simulink model "Clutchless_P2_Parallel"  (R2017b)
settings: Solver=FixedStepAuto  StartTime=0.0  StopTime=length(Speed)  FixedStep=0.01  MaxStep=0.01  RelTol=1e-3  EnableMultiTasking=on
PostLoadFcn:
  | , if any(exist('dsrtsu_mdlpostloadfcn', 'file') == [2, 3, 6]), try dsrtsu_mdlpostloadfcn('Execute', bdroot); catch fprintf('Error in PostLoadFcn (dsrtsu_mdlpostloadfcn) for model "%s":\n %s\n', bdroot, lasterr); end, end,
undefined symbols (not defined in the file): Actuators, APP1_OOR, APP2_OOR, APP_Mismatch, Brk_Flt, cal, Chassis, ClutchEngag, Clutchless_HSC, eng, Engine, EngineTorqueReal, EngOverTemp, ENGTRQ_MSMCH_Degraded_CP, ENGTRQ_MSMCH_ErrCritical_CP, ENGTRQ_MSMCH_LimpHome_CP, EngTrqMismatch, ess, ESSOverTemp, g, gb, Grade, KeyPos_Flt, lib_Actuators, lib_Chassis, lib_Clutchless_HSC, lib_EMachine_2017a, lib_Sensors_2017a, LossCAN, Machine, MCUOverTemp, mot, MotDirMismatch, motor_Trq, MotOverTemp, MotTrqMismatch, mph2ms, PRNDL_Flt, RegenFault, rho, Sensors, t_amb, time, tloop, veh, Vehicle
libraries: simulink x96, EC2_libraries x6, autolibmappedmotor x3, powerlib_meascontrol x2, CalculationGallon x1, lib_DCDC x1, lib_Differential x1, lib_HVESS x1, lib_Engine x1, lib_OBC x1, Scope_new x1, lib_Transmission x1
(part 6 of 10)

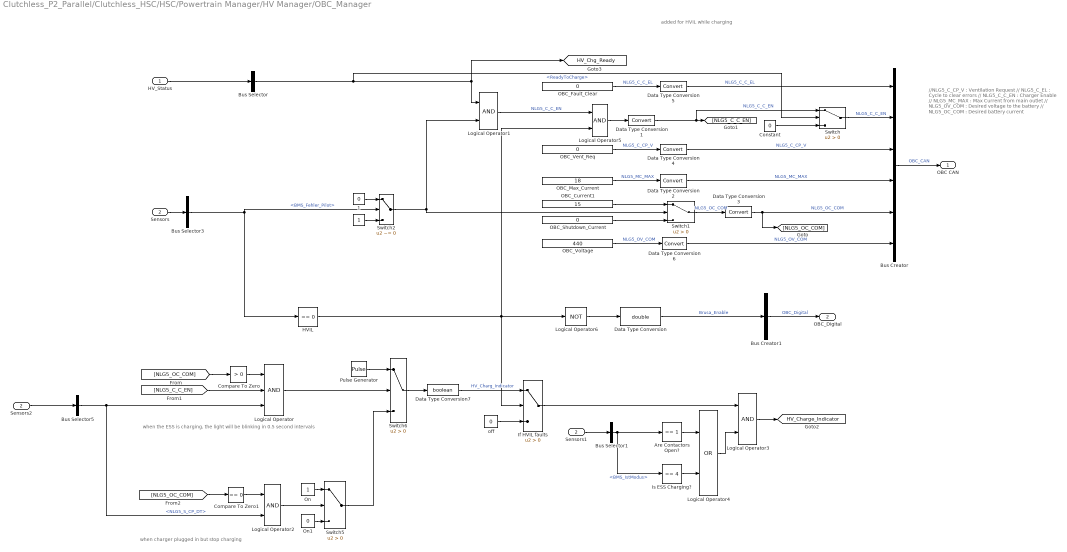
== system Clutchless_P2_Parallel/Clutchless_HSC/HSC/Powertrain Manager/HV Manager/OBC_Manager ==
  note: when the ESS is charging, the light will be blinking in 0.5 second intervals
  note: when charger plugged in but stop charging
  note: //NLG5_C_CP_V : Ventilation Request
      | // NLG5_C_EL : Cycle to clear errors
      | // NLG5_C_C_EN : Charger Enable
      | // NLG5_MC_MAX : Max Current from main outlet
      | // NLG5_OV_COM : Desired voltage to the battery
      | // NLG5_OC_COM : Desired battery current
  note: added for HVIL
      | while charging
  HV_Status : Inport
  Sensors : Inport  Port=2
  " " : Constant
  "   1" : Constant  Value=0
  Are Contactors Open? : simulink/Logic and Bit Operations/Compare To Constant  relop===  const=1  OutDataTypeStr=boolean
  Bus Creator : BusCreator  Inputs=6
  Bus Creator1 : BusCreator  Inputs=1
  Bus Selector : BusSelector  OutputSignals=ReadyToCharge
  Bus Selector1 : BusSelector  OutputSignals=from_CAN.fromHV_CAN.from_BMSHybrid.BMS_HYB_02.BMS_IstModus
  Bus Selector3 : BusSelector  OutputSignals=from_CAN.fromHV_CAN.from_BMSHybrid.BMS_HYB_02.BMS_Fehler_Pilot
  Bus Selector5 : BusSelector  OutputSignals=from_CAN.fromHV_CAN.from_OBC.NLG5_ST.NLG5_S_CP_DT
  Compare To Zero : simulink/Logic and Bit Operations/Compare To Zero  relop=>  OutDataTypeStr=boolean
  Compare To Zero1 : simulink/Logic and Bit Operations/Compare To Zero  relop===  OutDataTypeStr=boolean
  Constant : Constant  Value=0
  Data Type Conversion : DataTypeConversion  OutDataTypeStr=double
  Data Type Conversion{1..6} (6 alike) : DataTypeConversion
  Data Type Conversion7 : DataTypeConversion  OutDataTypeStr=boolean
  HVIL : simulink/Logic and Bit Operations/Compare To Constant  relop===  const=0  OutDataTypeStr=boolean
  If HVIL faults : Switch  Criteria=u2 > Threshold
  Is ESS Charging? : simulink/Logic and Bit Operations/Compare To Constant  relop===  const=4  OutDataTypeStr=boolean
  Logical Operator : Logic  Inputs=3  AllPortsSameDT=off  OutDataTypeStr=boolean
  Logical Operator{1..3,5} (4 alike) : Logic  AllPortsSameDT=off  OutDataTypeStr=boolean
  Logical Operator4 : Logic  Operator=OR  AllPortsSameDT=off  OutDataTypeStr=boolean
  Logical Operator6 : Logic  Operator=NOT  Inputs=3  AllPortsSameDT=off  OutDataTypeStr=boolean
  OBC_Current1 : Constant  Value=15
  OBC_Fault_Clear : Constant  Value=0
  OBC_Max_Current : Constant  Value=18
  OBC_Shutdown_Current : Constant  Value=0
  OBC_Vent_Req : Constant  Value=0
  OBC_Voltage : Constant  Value=440
  On : Constant
  On1 : Constant  Value=0
  Pulse Generator : DiscretePulseGenerator  PulseType=Time based  Period=1  PulseWidth=50
  Sensors1 : InportShadow  Port=2
  Sensors2 : InportShadow  Port=2
  Switch{,1,5..6} (4 alike) : Switch  Criteria=u2 > Threshold
  Switch2 : Switch  Criteria=u2 ~= 0
  off : Constant  Value=0
  OBC CAN : Outport
  OBC_Digital : Outport  Port=2
  tag scope: HV_Charge_Indicator=global, HV_Chg_Ready=global
  wires:
  Sensors2/1 -> Bus Selector5/1
  Switch/1 -> Bus Creator/2  "NLG5_C_C_EN"
  Constant/1 -> Switch/3
  Logical Operator6/1 -> Data Type Conversion/1
  Logical Operator5/1 -> Data Type Conversion1/1
  Logical Operator4/1 -> Logical Operator3/2
  Is ESS Charging?/1 -> Logical Operator4/2
  Bus Selector1/1 -> Are Contactors Open?/1, Is ESS Charging?/1  "<BMS_IstModus>"
  Are Contactors Open?/1 -> Logical Operator4/1
  Sensors1/1 -> Bus Selector1/1
  Logical Operator3/1 -> [HV_Charge_Indicator]
  off/1 -> If HVIL faults/3
  If HVIL faults/1 -> Logical Operator3/1
  HVIL/1 -> Logical Operator5/2, If HVIL faults/2, Logical Operator6/1
  "   1"/1 -> Switch2/1
  " "/1 -> Switch2/3
  Bus Creator1/1 -> OBC_Digital/1  "OBC_Digital"
  Data Type Conversion/1 -> Bus Creator1/1  "Brusa_Enable"
  Bus Selector3/1 -> Switch2/2, HVIL/1  "<BMS_Fehler_Pilot>"
  Bus Selector5/1 -> Logical Operator/3, Logical Operator2/2  "<NLG5_S_CP_DT>"
  Switch6/1 -> Data Type Conversion7/1
  Switch5/1 -> Switch6/3
  On1/1 -> Switch5/3
  On/1 -> Switch5/1
  Logical Operator2/1 -> Switch5/2
  Compare To Zero1/1 -> Logical Operator2/1
  [NLG5_OC_COM] -> Compare To Zero1/1
  Pulse Generator/1 -> Switch6/1
  Logical Operator/1 -> Switch6/2
  [NLG5_C_C_EN] -> Logical Operator/2
  Compare To Zero/1 -> Logical Operator/1
  [NLG5_OC_COM] -> Compare To Zero/1
  Sensors/1 -> Bus Selector3/1
  Bus Creator/1 -> OBC CAN/1  "OBC_CAN"
  HV_Status/1 -> Bus Selector/1
  Bus Selector/1 -> [HV_Chg_Ready], Logical Operator1/1, Switch/2  "<ReadyToCharge>"
  Switch2/1 -> Logical Operator1/2, Switch1/2
  Data Type Conversion2/1 -> Bus Creator/4  "NLG5_MC_MAX"
  Data Type Conversion5/1 -> Bus Creator/1  "NLG5_C_C_EL"
  Data Type Conversion4/1 -> Bus Creator/3  "NLG5_C_CP_V"
  Data Type Conversion6/1 -> Bus Creator/6  "NLG5_OV_COM"
  Data Type Conversion3/1 -> [NLG5_OC_COM], Bus Creator/5  "NLG5_OC_COM"
  OBC_Current1/1 -> Switch1/1
  OBC_Shutdown_Current/1 -> Switch1/3
  Data Type Conversion1/1 -> [NLG5_C_C_EN], Switch/1  "NLG5_C_C_EN"
  Logical Operator1/1 -> Logical Operator5/1  "NLG5_C_C_EN"
  Switch1/1 -> Data Type Conversion3/1  "NLG5_OC_COM"
  OBC_Vent_Req/1 -> Data Type Conversion4/1  "NLG5_C_CP_V"
  OBC_Fault_Clear/1 -> Data Type Conversion5/1  "NLG5_C_C_EL"
  OBC_Max_Current/1 -> Data Type Conversion2/1  "NLG5_MC_MAX"
  OBC_Voltage/1 -> Data Type Conversion6/1  "NLG5_OV_COM"
  Data Type Conversion7/1 -> If HVIL faults/1  "HV_Charg_Indicator"

== system Clutchless_P2_Parallel/Clutchless_HSC/HSC/Powertrain Manager/Thermal Manager/Cooling Fan Manger ==
  Temp : Inport
  Bus Selector : BusSelector  OutputSignals=Temp_Signals.EngCltTmp,Temp_Signals.BMS_Temperatur,Temp_Signals.INV_ElectricMachineTemperature,Temp_Signals.INV_InverterTemperature,VehSpdAvgDrvn,Component_State.SysPwrMd
  Constant : Constant  Value=0
  ESSTargTemp : RelationalOperator  OutDataTypeStr=boolean  RndMeth=Nearest
  EnTargTemp : RelationalOperator  OutDataTypeStr=boolean  RndMeth=Nearest
  EnTargTemp1 : RelationalOperator  Operator=>  OutDataTypeStr=boolean  RndMeth=Nearest
  Fan_Disable : Constant  Value=0
  Fan_Enable : Constant
  Fan_EngTempThrshld : Constant  Value=100
  Fan_EssTempThrshld : Constant  Value=25
  Fan_MCUTempThrshld : Constant  Value=35
  Fan_MotTempThrshld : Constant  Value=35
  Fan_VehSpdThrshld : Constant  Value=10
  InvTargTemp : RelationalOperator  OutDataTypeStr=boolean  RndMeth=Nearest
  InvTargTemp1 : RelationalOperator  Operator=<=  OutDataTypeStr=boolean  RndMeth=Nearest
  Logical Operator : Logic  Operator=OR  Inputs=4  AllPortsSameDT=off  OutDataTypeStr=boolean
  Logical Operator1 : Logic  AllPortsSameDT=off  OutDataTypeStr=boolean
  Logical Operator2 : Logic  AllPortsSameDT=off  OutDataTypeStr=boolean
  MorTargTemp : RelationalOperator  OutDataTypeStr=boolean  RndMeth=Nearest
  Switch : Switch  Criteria=u2 ~= 0
  Fan_control : Outport
  wires:
  Fan_VehSpdThrshld/1 -> InvTargTemp1/2
  Fan_MCUTempThrshld/1 -> InvTargTemp/2
  Fan_MotTempThrshld/1 -> MorTargTemp/2
  Fan_EssTempThrshld/1 -> ESSTargTemp/2
  Fan_EngTempThrshld/1 -> EnTargTemp/2
  InvTargTemp1/1 -> Logical Operator1/2
  Bus Selector/5 -> InvTargTemp1/1  "<VehSpdAvgDrvn>"
  Logical Operator/1 -> Logical Operator1/1
  InvTargTemp/1 -> Logical Operator/4
  MorTargTemp/1 -> Logical Operator/3
  ESSTargTemp/1 -> Logical Operator/2
  EnTargTemp/1 -> Logical Operator/1
  Bus Selector/4 -> InvTargTemp/1  "<INV_InverterTemperature>"
  Bus Selector/3 -> MorTargTemp/1  "<INV_ElectricMachineTemperature>"
  Bus Selector/2 -> ESSTargTemp/1  "<BMS_Temperatur>"
  Bus Selector/1 -> EnTargTemp/1  "<EngCltTmp>"
  Fan_Enable/1 -> Switch/1
  Fan_Disable/1 -> Switch/3
  Switch/1 -> Fan_control/1
  Temp/1 -> Bus Selector/1
  Logical Operator2/1 -> Switch/2
  Logical Operator1/1 -> Logical Operator2/1
  EnTargTemp1/1 -> Logical Operator2/2
  Bus Selector/6 -> EnTargTemp1/1  "<SysPwrMd>"
  Constant/1 -> EnTargTemp1/2

== system Clutchless_P2_Parallel/Clutchless_HSC/HSC/Powertrain Manager/Thermal Manager/ESS Pump Manger ==
  note: If ESS temp>35°，enable pump100 and cooling fan and 2-way valve then enable AC-compressor
      |
      | If 35°>ESStemp≥23°，enable pump100 and cooling fan
      |
      | If 23°>ESS temp disable
      |
      | If 15°>ESS temp, enable heat coolant
  ESS_temp : Inport
  Bus Creator : BusCreator  Inputs=4
  Bus Selector : BusSelector  OutputSignals=Temp_Signals.BMS_Temperatur,Component_State.SysPwrMd
  Chart1 : Stateflow chart  TreatAsAtomicUnit=on
  ESS_Comp_TempThrs : Constant  Value=35
  ESS_Temp_State_1_Thrs : Constant  Value=15
  ESS_Temp_State_2_Thrs : Constant  Value=25
  ESS_Temp_State_3_Thrs : Constant  Value=35
  ESS_Thermal_Control : Outport
  wires:
  Bus Creator/1 -> ESS_Thermal_Control/1
  ESS_Comp_TempThrs/1 -> Chart1/5(ESS_Comp_TempThrs)
  ESS_Temp_State_3_Thrs/1 -> Chart1/4(ESS_Temp_State_3_Thrs)
  ESS_Temp_State_2_Thrs/1 -> Chart1/3(ESS_Temp_State_2_Thrs)
  ESS_Temp_State_1_Thrs/1 -> Chart1/2(ESS_Temp_State_1_Thrs)
  Chart1/3(ESS_val) -> Bus Creator/3  "ESS_val"
  Chart1/2(ESS_pump_control) -> Bus Creator/2  "ESS_pump_control"
  Chart1/1(ESS_comp) -> Bus Creator/1  "ESS_comp"
  Bus Selector/1 -> Chart1/1(ESS_temp), Chart1/6(ESS_CltTemp)  "<BMS_Temperatur>"
  ESS_temp/1 -> Bus Selector/1
  Chart1/4(ESS_comp_Enable) -> Bus Creator/4  "ESS_Comp_Enable"
  Bus Selector/2 -> Chart1/7(SysPowMod)  "<SysPwrMd>"

== system Clutchless_P2_Parallel/Clutchless_HSC/HSC/Powertrain Manager/Thermal Manager/MotInv Pump Manger ==
  MotInv_temp : Inport
  Bus Selector : BusSelector  OutputSignals=Temp_Signals.INV_ElectricMachineTemperature,Temp_Signals.INV_InverterTemperature,Component_State.SysPwrMd
  MCUPump_Manager : Stateflow chart  TreatAsAtomicUnit=on
  MCU_Temp_State_1_Thrs : Constant  Value=30
  MCU_Temp_State_2_Thrs : Constant  Value=50
  Mot_Temp_State_1_Thrs : Constant  Value=30
  Mot_Temp_State_2_Thrs1 : Constant  Value=45
  MotInvpump_control : Outport
  wires:
  MCU_Temp_State_2_Thrs/1 -> MCUPump_Manager/6(Mot_Temp_State_2_Thrs)
  Mot_Temp_State_2_Thrs1/1 -> MCUPump_Manager/5(MCU_Temp_State_2_Thrs)
  Mot_Temp_State_1_Thrs/1 -> MCUPump_Manager/3(MCU_Temp_State_1_Thrs)
  MCU_Temp_State_1_Thrs/1 -> MCUPump_Manager/4(Mot_Temp_State_1_Thrs)
  Bus Selector/2 -> MCUPump_Manager/2(MCU_temp)  "<INV_InverterTemperature>"
  Bus Selector/1 -> MCUPump_Manager/1(Motor_temp)  "<INV_ElectricMachineTemperature>"
  MotInv_temp/1 -> Bus Selector/1
  Bus Selector/3 -> MCUPump_Manager/7(SysPowMod)  "<SysPwrMd>"
  MCUPump_Manager/1(MotInvpump_control) -> MotInvpump_control/1

== system Clutchless_P2_Parallel/Clutchless_HSC/HSC/Powertrain Manager/Torque Distribution/AxlTrq_to_EngTrq ==
  note: //From engine axle torque to engine torque//
  note: check this rate limiter
  In1 : Inport
  Compare To Constant : simulink/Logic and Bit Operations/Compare To Constant  relop===  const=0  OutDataTypeStr=boolean
  Constant1 : Constant  Value=max(gb.plant.init.ratio.map)
  Constant5 : Constant  Value=fd.plant.init.ratio
  Divide1 : Product  Inputs=*//
  Ground : Ground  Commented=on
  Rate Limiter : RateLimiter  RisingSlewLimit=1000  FallingSlewLimit=-2000
  Rate Limiter1 : RateLimiter  Commented=on  RisingSlewLimit=Engine.trq_uprate  FallingSlewLimit=Engine.trq_derate
  Ratio Filter : Subsystem
  Switch : Switch  Criteria=u2 > Threshold
  Terminator : Terminator  Commented=on
  Out1 : Outport
  wires:
  Ground/1 -> Rate Limiter1/1
  Rate Limiter1/1 -> Terminator/1
  Ratio Filter/1(Filtered_Ratio) -> Compare To Constant/1, Switch/3
  Rate Limiter/1 -> Out1/1
  Switch/1 -> Divide1/3
  Constant1/1 -> Switch/1
  Compare To Constant/1 -> Switch/2
  [TransRatio] -> Ratio Filter/1(Ratio)
  Divide1/1 -> Rate Limiter/1
  Constant5/1 -> Divide1/2
  In1/1 -> Divide1/1

== system Clutchless_P2_Parallel/Clutchless_HSC/HSC/Powertrain Manager/Torque Distribution/AxlTrq_to_MotTrq ==
  In1 : Inport
  AxlTrq_to_MtrTrq2 : Subsystem
  MotTrq_LowLim : Constant  Value=-250
  MotTrq_UpLim : Constant  Value=325
  Saturation Dynamic : simulink/Discontinuities/Saturation Dynamic  OutMin=[]  OutMax=[]  OutDataTypeStr=Inherit: Same as second input  OutDataType=fixdt(1, 16)  OutScaling=2^-10  DoSatur=off
  electric machine filter : Subsystem
  Out1 : Outport
  wires:
  Saturation Dynamic/1 -> Out1/1  "MtrTrqCmd_AftSat"
  electric machine filter/1(filtered) -> Saturation Dynamic/2  "MotTrqCmd_BefSat"
  AxlTrq_to_MtrTrq2/1(MtrTrqCmd) -> electric machine filter/1(trq)  "MtrTrqCmd"
  In1/1 -> AxlTrq_to_MtrTrq2/1(In1)
  MotTrq_UpLim/1 -> Saturation Dynamic/1
  MotTrq_LowLim/1 -> Saturation Dynamic/3

== system Clutchless_P2_Parallel/Clutchless_HSC/HSC/Powertrain Manager/Torque Distribution/Rate Limiter Motor1 ==
  In1 : Inport
  Compare To Constant : simulink/Logic and Bit Operations/Compare To Constant  relop===  const=4  OutDataTypeStr=boolean
  Derate_CDCS Mode : Constant  Value=-80
  Derate_Sports Mode : Constant  Value=-150
  Rate Limiter Dynamic : simulink/Discontinuities/Rate Limiter Dynamic
      settings: SourceProductName=Simulink
  Switch : Switch  Criteria=u2 > Threshold
  Switch1 : Switch  Criteria=u2 > Threshold
  Uprate_CDCS Mode : Constant  Value=80
  Uprate_Sports Mode : Constant  Value=100
  Out1 : Outport
  wires:
  Compare To Constant/1 -> Switch/2, Switch1/2
  [mode] -> Compare To Constant/1
  Derate_Sports Mode/1 -> Switch1/1
  Derate_CDCS Mode/1 -> Switch1/3
  Switch1/1 -> Rate Limiter Dynamic/3
  Uprate_CDCS Mode/1 -> Switch/3
  Switch/1 -> Rate Limiter Dynamic/1
  Uprate_Sports Mode/1 -> Switch/1
  Rate Limiter Dynamic/1 -> Out1/1
  In1/1 -> Rate Limiter Dynamic/2

== system Clutchless_P2_Parallel/Clutchless_HSC/HSC/Powertrain Manager/Torque Distribution/RegTrqLimit ==
  MotTrqCmd : Inport
  RPM : Inport  Port=2
  Compare To Constant : simulink/Logic and Bit Operations/Compare To Constant  relop=<=  const=0  OutDataTypeStr=boolean
  Divide : Product  Inputs=**
  Regen Trq Derating : Lookup_n-D  NumberOfTableDimensions=1  BreakpointsForDimension1=[0,200,600,800,1000]  Table=[0,0,0,0.8,1]  ExtrapMethod=Clip  UseLastTableValue=on  InternalRulePriority=Speed  RndMeth=Simplest  InputSameDT=on
  Regen Trq Derating1 : Lookup_n-D  Commented=on  NumberOfTableDimensions=1  BreakpointsForDimension1=[0 200 600 800 1000 1200 12000]  Table=[0 0.05 0.5 0.8 0.95 1 1]  ExtrapMethod=Clip  UseLastTableValue=on  InternalRulePriority=Speed  RndMeth=Simplest  InputSameDT=on
  Switch2 : Switch  Criteria=u2 > Threshold
  Out1 : Outport
  wires:
  Regen Trq Derating/1 -> Divide/1
  Divide/1 -> Switch2/1
  Compare To Constant/1 -> Switch2/2
  MotTrqCmd/1 -> Switch2/3, Divide/2, Compare To Constant/1  "MotTrqCmdIn"
  Switch2/1 -> Out1/1  "MotTrqCmdOut"
  RPM/1 -> Regen Trq Derating/1

== system Clutchless_P2_Parallel/Clutchless_HSC/HSC/Powertrain Manager/Torque Distribution/Select_APP ==
  APP_Select : Constant  Value=0
  Data Type Conversion10 : DataTypeConversion  OutDataTypeStr=boolean
  Derate_APP : Constant  Value=-100
  Rate Limiter Dynamic : simulink/Discontinuities/Rate Limiter Dynamic
      settings: SourceProductName=Simulink
  Switch1 : Switch  Criteria=u2 > Threshold
  Uprate_APP : Constant  Value=80
  EngAppReq : Outport
  wires:
  [EngAppReq] -> Switch1/3
  [AccPos_Perc] -> Switch1/1
  Data Type Conversion10/1 -> Switch1/2
  APP_Select/1 -> Data Type Conversion10/1
  Switch1/1 -> Rate Limiter Dynamic/2  "EngAppReq"
  Rate Limiter Dynamic/1 -> EngAppReq/1  "EngAppReq_Limited"
  Uprate_APP/1 -> Rate Limiter Dynamic/1
  Derate_APP/1 -> Rate Limiter Dynamic/3

== system Clutchless_P2_Parallel/Clutchless_HSC/HSC/Powertrain Manager/Torque Distribution/Sport Mode Enable ==
  In1 : Inport
  Bus Selector5 : BusSelector  OutputSignals=from_Analog.Sport_Mode_SW
  Compare To Constant : simulink/Logic and Bit Operations/Compare To Constant  relop===  const=2  OutDataTypeStr=boolean
  Override Sport Switch : Subsystem
  Sports Mode Logic : Stateflow chart  TreatAsAtomicUnit=on
  Out1 : Outport
  wires:
  In1/1 -> Bus Selector5/1
  Bus Selector5/1 -> Sports Mode Logic/1(Voltage_Input)  "<Sport_Mode_SW>"
  Sports Mode Logic/1(Driver_Mode) -> Compare To Constant/1
  Compare To Constant/1 -> Override Sport Switch/1(In1)
  Override Sport Switch/1(Out1) -> Out1/1

== system Clutchless_P2_Parallel/Clutchless_HSC/HSC/Powertrain Manager/Torque Distribution/Subsystem1 ==
  SoC : Inport
  CS_On : Inport  Port=2
  Constant : Constant
  Sample and Hold1 : dspsigops/Sample and Hold  trig=Rising edge  initCond=0  latchinput=off
  Switch : Switch  Criteria=u2 > Threshold
  Faked_SoC : Outport
  wires:
  SoC/1 -> Sample and Hold1/1
  CS_On/1 -> Switch/2, Sample and Hold1/Trigger
  Switch/1 -> Faked_SoC/1
  Sample and Hold1/1 -> Switch/1
  Constant/1 -> Switch/3

== system Clutchless_P2_Parallel/Clutchless_HSC/HSC/Powertrain Manager/Torque Distribution/Supervisory  Control  Logic/VehReady.CD_Mode.Brake_mode.MotTrqCalc1 ==
  note: Regenerative braking:
      | Regenerative braking should be allowed under specific chassis speed:
      | chas_spd_below_no_regen= 1.5;
      | chas_spd_above_full_regen = 3;
      | ess_soc_above_regen_forbidden = .92;  % ESS SOC above which regen braking is forbidden
      | ess_soc_above_regen_allowed = .9;% ESS SOC above which regen braking is allowed
  BPP : Inport
  VehSpd : Inport  Port=2
  ShftLvrPos : Inport  Port=3
  MotSpeed : Inport  Port=4
  TransRatio : Inport  Port=5
  IntdAxleTrq : Inport  Port=6
  f : TriggerPort  TriggerType=function-call  VariantControl=Variant
      settings: CopyFcn=Stateflow.SLINSF.SimulinkMan.removeBlockPreDeleteFcn  PreDeleteFcn=Stateflow.SLINSF.SimulinkMan.unsafePredeleteFcn
  "% to 1 " : Gain  Gain=1/100
  Constant : Constant  Value=0
  Constant1 : Constant  Value=0
  Constant2 : Constant  Value=fd.plant.init.ratio
  Divide : Product  Inputs=***
  Divide2 : Product  Inputs=***
  Index Vector : MultiPortSwitch  DataPortOrder=Zero-based contiguous  Inputs=5  zeroidx=on
  MinMax : MinMax  Function=max  Inputs=2
  Peak trq max - Regen : Lookup  InputValues=mot.plant.init.regen.trq_max.idx1_spd  Table=mot.plant.init.regen.trq_max.map  LookUpMeth=Interpolation-Use End Values  SaturateOnIntegerOverflow=on
  Regen Trq Derating2 : Lookup_n-D  NumberOfTableDimensions=1  BreakpointsForDimension1=[0 10 11 200]  Table=[0 0.5 1 1]  ExtrapMethod=Clip  UseLastTableValue=on  InternalRulePriority=Speed  RndMeth=Simplest  InputSameDT=on
  Regen_derat_overri : Constant  Value=0
  Regen_derat_value : Constant  Value=0.5
  Switch : Switch  Criteria=u2 > Threshold
  limit to -200Nm : Saturate  UpperLimit=0  LowerLimit=-200
  T : Outport
  wires:
  MinMax/1 -> [TrqCalc]
  IntdAxleTrq/1 -> MinMax/1
  Regen_derat_value/1 -> Switch/1
  Switch/1 -> Divide/3
  Regen_derat_overri/1 -> Switch/2
  Regen Trq Derating2/1 -> Switch/3
  Divide2/1 -> MinMax/2  "motor"
  TransRatio/1 -> Divide2/3
  limit to -200Nm/1 -> Divide2/2
  Constant2/1 -> Divide2/1
  Peak trq max - Regen/1 -> Divide/2
  MotSpeed/1 -> Peak trq max - Regen/1  "RPM"
  [TrqCalc] -> Index Vector/5  "N"
  Constant1/1 -> Index Vector/3  "P"
  Constant/1 -> Index Vector/2  "Between Ranges"
  Index Vector/1 -> T/1
  [TrqCalc] -> Index Vector/6  "D"
  [TrqCalc] -> Index Vector/4  "R"
  ShftLvrPos/1 -> Index Vector/1
  VehSpd/1 -> Regen Trq Derating2/1
  Divide/1 -> limit to -200Nm/1
  "% to 1 "/1 -> Divide/1
  BPP/1 -> "% to 1 "/1

== system Clutchless_P2_Parallel/Clutchless_HSC/HSC/Powertrain Manager/Torque Distribution/Supervisory  Control  Logic/VehReady.CD_Mode.Brake_mode.MotTrqCalc2 ==
  note: Regenerative braking:
      | Regenerative braking should be allowed under specific chassis speed:
      | chas_spd_below_no_regen= 1.5;
      | chas_spd_above_full_regen = 3;
      | ess_soc_above_regen_forbidden = .92;  % ESS SOC above which regen braking is forbidden
      | ess_soc_above_regen_allowed = .9;% ESS SOC above which regen braking is allowed
  ShftLvrPos : Inport
  TransRatio : Inport  Port=2
  f : TriggerPort  TriggerType=function-call  VariantControl=Variant
      settings: CopyFcn=Stateflow.SLINSF.SimulinkMan.removeBlockPreDeleteFcn  PreDeleteFcn=Stateflow.SLINSF.SimulinkMan.unsafePredeleteFcn
  Constant : Constant  Value=0
  Constant1 : Constant  Value=0
  Constant2 : Constant  Value=fd.plant.init.ratio
  Divide2 : Product  Inputs=***
  Idle_torque_Regen : Constant  Value=0
  Index Vector : MultiPortSwitch  DataPortOrder=Zero-based contiguous  Inputs=5  zeroidx=on
  T : Outport
  wires:
  Idle_torque_Regen/1 -> Divide2/2
  Divide2/1 -> [TrqCalc]  "motor"
  TransRatio/1 -> Divide2/3
  Constant2/1 -> Divide2/1
  [TrqCalc] -> Index Vector/5  "N"
  Constant1/1 -> Index Vector/3  "P"
  Constant/1 -> Index Vector/2  "Between Ranges"
  Index Vector/1 -> T/1
  [TrqCalc] -> Index Vector/6  "D"
  [TrqCalc] -> Index Vector/4  "R"
  ShftLvrPos/1 -> Index Vector/1

== system Clutchless_P2_Parallel/Clutchless_HSC/HSC/Powertrain Manager/Torque Distribution/Supervisory  Control  Logic/VehReady.CD_Mode.Drive_mode.EngTrq2EngApp ==
  Trq : Inport
  TransRatio : Inport  Port=2
  f : TriggerPort  TriggerType=function-call  VariantControl=Variant
      settings: CopyFcn=Stateflow.SLINSF.SimulinkMan.removeBlockPreDeleteFcn  PreDeleteFcn=Stateflow.SLINSF.SimulinkMan.unsafePredeleteFcn
  0-100% : Saturate  UpperLimit=100  LowerLimit=0
  Compare To Constant : simulink/Logic and Bit Operations/Compare To Constant  relop===  const=0  OutDataTypeStr=boolean
  Constant1 : Constant  Value=eps
  Constant5 : Constant  Value=fd.plant.init.ratio
  Divide1 : Product  Inputs=*//
  EngTrq2EngAPP : Lookup_n-D  NumberOfTableDimensions=1  BreakpointsForDimension1=[0:1:230]  Table="[-0.950562242591810\t-0.861179388327002\t-0.757792747831397\t-0.640901927898975\t-0.511000095283862\t-0.368573976700328\t-0.214103858822793\t-0.0480635882858183\t0.129079428315885\t0.316864224427463\t0.514836273533913\t0.722547489160089\t0.939556224870697\t1.16542727427030\t1.39973187100331\t1.64204768875400\t1.89195884124648\t2.14905588224475\t2.41293580555262\t2.68320204501379\t2.95946447451180\t3.24133940797003\t3.52844959935174\t3.82042424266002\t4.11689897193784\t4.41751586126800\t4.72192342477317\t5.02977661661586\t5.34073683099846\t5.65447190216317\t5.97065610439209\t6.28897015200715\t6.60910119937013\t6.93074284088268\t7.25359511098630\t7.57736448416234\t7.90176387493200\t8.22651263785634\t8.55133656753627\t8.87596789861257\t9.20014530576584\t9.52361390371657\t9.84612524722509\t10.1674373310916\t10.4873145901561\t10.8055278992985\t11.1218545734385\t11.4360783675358\t11.7479894765898\t12.0573845356398\t12.3640666197649\t12.6678452440843\t12.9685363637566\t13.2659623739808\t13.5599521099953\t13.8503408470787\t14.1369703005491\t14.4196886257647\t14.6983504181235\t14.9728167130634\t15.2429549860620\t15.5086391526369\t15.7697495683456\t16.0261730287853\t16.2778027695931\t16.5245384664460\t16.7662862350608\t17.0029586311942\t17.2344746506427\t17.4607597292427\t17.6817457428705\t17.8973710074422\t18.1075802789137\t18.3123247532808\t18.5115620665792\t18.7052562948843\t18.8933779543117\t19.0759040010164\t19.2528178311935\t19.4241092810781\t19.5897746269448\t19.7498165851084\t19.9042443119232\t20.0530734037837\t20.1963258971241\t20.3340302684184\t20.4662214341804\t20.5929407509641\t20.7142360153630\t20.8301614640105\t20.9407777735800\t21.0461520607847\t21.1463578823776\t21.2414752351516\t21.3315905559394\t21.4167967216136\t21.4971930490867\t21.5728852953111\t21.6439856572787\t21.7106127720217\t21.7728917166119\t21.8309540081611\t21.8849376038208\t21.9349869007824\t21.9812527362772\t22.0238923875764\t22.0630695719909\t22.0989544468717\t22.1317236096093\t22.1615600976344\t22.1886533884173\t22.2131993994684\t22.2354004883376\t22.2554654526151\t22.2736095299306\t22.2900543979538\t22.3050281743942\t22.3187654170013\t22.3315071235641\t22.3435007319120\t22.3550001199137\t22.3662656054781\t22.3775639465539\t22.3891683411296\t22.4013584272335\t22.4144202829338\t22.4286464263386\t22.4443358155959\t22.4617938488934\t22.4813323644587\t22.5032696405595\t22.5279303955028\t22.5556457876361\t22.5867534153463\t22.6215973170604\t22.6605279712450\t22.7039022964069\t22.7520836510924\t22.8054418338880\t22.8643530834197\t22.9292000783536\t23.0003719373956\t23.0782642192915\t23.1632789228268\t23.2558244868269\t23.3563157901571\t23.4651741517227\t23.5828273304686\t23.7097095253797\t23.8462613754808\t23.9929299598362\t24.1501687975506\t24.3184378477682\t24.4982035096730\t24.6899386224892\t24.8941224654804\t25.1112407579505\t25.3417856592430\t25.5862557687413\t25.8451561258686\t26.1189982100880\t26.4082999409026\t26.7135856778550\t27.0353862205281\t27.3742388085443\t27.7306871215661\t28.1052812792955\t28.4985778414748\t28.9111398078859\t29.3435366183506\t29.7963441527305\t30.2701447309271\t30.7655271128819\t31.2830864985759\t31.8234245280303\t32.3871492813060\t32.9748752785038\t33.5872234797643\t34.2248212852680\t34.8883025352352\t35.5783075099261\t36.2954829296408\t37.0404819547192\t37.8139641855409\t38.6165956625258\t39.4490488661331\t40.3120027168621\t41.2061425752523\t42.1321602418824\t43.0907539573713\t44.0826284023780\t45.1084946976008\t46.1690704037782\t47.2650795216887\t48.3972524921501\t49.5663261960208\t50.7730439541983\t52.0181555276205\t53.3024171172650\t54.6265913641491\t55.9914473493301\t57.3977605939052\t58.8463130590113\t60.3378931458253\t61.8732956955639\t63.4533219894835\t65.0787797488808\t66.7504831350916\t68.4692527494924\t70.2359156334991\t72.0513052685674\t73.9162615761929\t75.8316309179113\t77.7982660952979\t79.8170263499681\t81.8887773635766\t84.0143912578187\t86.1947465944290\t88.4307283751822\t90.7232280418928\t93.0731434764153\t95.4813790006436\t97.9488453765121\t100\t100\t100\t100\t100\t100\t100\t100]"  ExtrapMethod=Clip  UseLastTableValue=on  InternalRulePriority=Speed  RndMeth=Simplest  InputSameDT=on
  Switch : Switch  Criteria=u2 > Threshold
  APP : Outport
  wires:
  EngTrq2EngAPP/1 -> 0-100%/1  "EngTrq2EngAPP"
  0-100%/1 -> APP/1
  TransRatio/1 -> Compare To Constant/1, Switch/3
  Divide1/1 -> EngTrq2EngAPP/1  "CDEngTrqCmd"
  Switch/1 -> Divide1/3
  Constant1/1 -> Switch/1
  Compare To Constant/1 -> Switch/2
  Constant5/1 -> Divide1/2
  Trq/1 -> Divide1/1  "CDEngAxlTrqCmd"

== system Clutchless_P2_Parallel/Clutchless_HSC/HSC/Powertrain Manager/Torque Distribution/Supervisory  Control  Logic/VehReady.CD_Mode.Drive_mode.EngTrqCalc ==
  EngSpeed : Inport
  APP : Inport  Port=2
  VehSpd : Inport  Port=3
  ShftLvrPos : Inport  Port=4
  DrvIntdAxleTrq : Inport  Port=5
  TransRatio : Inport  Port=6
  f : TriggerPort  TriggerType=function-call  VariantControl=Variant
      settings: CopyFcn=Stateflow.SLINSF.SimulinkMan.removeBlockPreDeleteFcn  PreDeleteFcn=Stateflow.SLINSF.SimulinkMan.unsafePredeleteFcn
  APP Derating : Lookup_n-D  NumberOfTableDimensions=1  BreakpointsForDimension1=[0 1 2 3 ]  Table=[0 0 0.1 1]  ExtrapMethod=Clip  UseLastTableValue=on  InternalRulePriority=Speed  RndMeth=Simplest  InputSameDT=on
  Constant : Constant  Value=0
  Constant1 : Constant  Value=0
  Constant3 : Constant  Value=fd.plant.init.ratio
  Divide : Product  Inputs=***
  Divide2 : Product  Inputs=***
  EngOptmTrq_Scaled_30% : Lookup_n-D  NumberOfTableDimensions=1  BreakpointsForDimension1=[1550 1650 1850 2050 2350 2650 2950 3150 3250 3350]  Table="[46.2063   52.0871   54.1987   55.8983   54.8577   54.0526   53.4113   54.5674   57.2958   59.8613]"  ExtrapMethod=Clip  UseLastTableValue=on  InternalRulePriority=Speed  RndMeth=Simplest  InputSameDT=on
  MinMax : MinMax  Inputs=2
  Scope : Scope  NumInputPorts=2
  Shifter : MultiPortSwitch  DataPortOrder=Zero-based contiguous  Inputs=5  zeroidx=on
  VehSpd Derating : Lookup_n-D  NumberOfTableDimensions=1  BreakpointsForDimension1=[0 5 10 20]  Table=[0 0.2 0.8 1]  ExtrapMethod=Clip  UseLastTableValue=on  InternalRulePriority=Speed  RndMeth=Simplest  InputSameDT=on
  Trq : Outport
  EngTrqAct : Outport  Port=2
  wires:
  MinMax/1 -> [TrqCalc]  "EngAxlTrqReq_CD"
  DrvIntdAxleTrq/1 -> Scope/2, MinMax/1  "driver"
  TransRatio/1 -> Divide2/3
  Divide2/1 -> Scope/1, EngTrqAct/1, MinMax/2  "EngAxlTrqAvl_CD"
  Divide/1 -> Divide2/2
  Constant3/1 -> Divide2/1
  Shifter/1 -> Trq/1
  [TrqCalc] -> Shifter/5  "N"
  Constant1/1 -> Shifter/3  "P"
  Constant/1 -> Shifter/2  "Between Ranges"
  [TrqCalc] -> Shifter/6  "D"
  [TrqCalc] -> Shifter/4  "R"
  ShftLvrPos/1 -> Shifter/1
  VehSpd Derating/1 -> Divide/3  "VehSpeedDerating_CD"
  VehSpd/1 -> VehSpd Derating/1
  APP Derating/1 -> Divide/2  "APPDerating_CD"
  APP/1 -> APP Derating/1
  EngSpeed/1 -> EngOptmTrq_Scaled_30%/1
  EngOptmTrq_Scaled_30%/1 -> Divide/1  "EngTrqAvl_CD"

== system Clutchless_P2_Parallel/Clutchless_HSC/HSC/Powertrain Manager/Torque Distribution/Supervisory  Control  Logic/VehReady.CD_Mode.Drive_mode.MotTrqCalc2 ==
  APP : Inport
  ShftLvrPos : Inport  Port=2
  DrvIntdAxleTrq : Inport  Port=3
  TransRatio : Inport  Port=4
  EngTrqAct : Inport  Port=5
  f : TriggerPort  TriggerType=function-call  VariantControl=Variant
      settings: CopyFcn=Stateflow.SLINSF.SimulinkMan.removeBlockPreDeleteFcn  PreDeleteFcn=Stateflow.SLINSF.SimulinkMan.unsafePredeleteFcn
  0-100% : Saturate  UpperLimit=100  LowerLimit=0
  Constant : Constant  Value=0
  Constant1 : Constant  Value=0
  Constant4 : Constant  Value=fd.plant.init.ratio
  Divide2 : Product  Inputs=***
  Index Vector : MultiPortSwitch  DataPortOrder=Zero-based contiguous  Inputs=5  zeroidx=on
  MinMax : MinMax  Inputs=2
  No Torque : Constant  Value=0
  Sum : Sum  Inputs=+-
  Switch : Switch  Criteria=u2 > Threshold  Threshold=3.5
  drvAPP2CmbTrq : Lookup_n-D  NumberOfTableDimensions=1  BreakpointsForDimension1=[0,1,2,3,4,5,6,7,8,9,10,11,12,13,14,15,16,17,18,19,20,21,22,23,24,25,26,27,28,29,30,31,32,33,34,35,36,37,38,39,40,41,42,43,44,45,46,47,48,49,50,51,52,53,54,55,56,57,58,59,60,70,80,90,100]  Table=[10.5,10.5,10.5,10.5,11,11,11.5,11.5,12,12,12,15,20,25,30,35,40,45,50,55,65,75,85,95,105,115,116,117,118,119,120,121,122,123,124,125,135,140,145,150,150,150,155,160,165,170,175,180,190,195,200,205,210,215,220,225,230,235,240,245,250,275,300,325,350]  ExtrapMethod=Clip  UseLastTableValue=on  InternalRulePriority=Speed  RndMeth=Simplest  InputSameDT=on
  MotTrq : Outport
  wires:
  Sum/1 -> MinMax/1
  EngTrqAct/1 -> Sum/2
  DrvIntdAxleTrq/1 -> Sum/1  "DrvIntdAxleTrq_CD"
  drvAPP2CmbTrq/1 -> Divide2/3
  MinMax/1 -> [TrqCalc]  "MotAxlTrqReq_CD"
  No Torque/1 -> Switch/3
  TransRatio/1 -> Divide2/1
  Switch/1 -> MinMax/2  "MotAxlTrqAvl_CD"
  Divide2/1 -> Switch/1
  APP/1 -> drvAPP2CmbTrq/1, 0-100%/1
  Constant4/1 -> Divide2/2
  Index Vector/1 -> MotTrq/1
  [TrqCalc] -> Index Vector/5  "N"
  Constant1/1 -> Index Vector/3  "P"
  Constant/1 -> Index Vector/2  "Between Ranges"
  [TrqCalc] -> Index Vector/6  "D"
  [TrqCalc] -> Index Vector/4  "R"
  ShftLvrPos/1 -> Index Vector/1
  0-100%/1 -> Switch/2

== system Clutchless_P2_Parallel/Clutchless_HSC/HSC/Powertrain Manager/Torque Distribution/Supervisory  Control  Logic/VehReady.CS_Mode.Engine_Charge.Brake_mode1.MotTrqCalc1 ==
  note: Regenerative braking:
      | Regenerative braking should be allowed under specific chassis speed:
      | chas_spd_below_no_regen= 1.5;
      | chas_spd_above_full_regen = 3;
      | ess_soc_above_regen_forbidden = .92;  % ESS SOC above which regen braking is forbidden
      | ess_soc_above_regen_allowed = .9;% ESS SOC above which regen braking is allowed
  BPP : Inport
  VehSpd : Inport  Port=2
  ShftLvrPos : Inport  Port=3
  MotSpeed : Inport  Port=4
  TransRatio : Inport  Port=5
  IntdAxleTrq : Inport  Port=6
  f : TriggerPort  TriggerType=function-call  VariantControl=Variant
      settings: CopyFcn=Stateflow.SLINSF.SimulinkMan.removeBlockPreDeleteFcn  PreDeleteFcn=Stateflow.SLINSF.SimulinkMan.unsafePredeleteFcn
  "% to 1 " : Gain  Gain=1/100
  Constant : Constant  Value=0
  Constant1 : Constant  Value=0
  Constant2 : Constant  Value=fd.plant.init.ratio
  Divide : Product  Inputs=***
  Divide2 : Product  Inputs=***
  Index Vector : MultiPortSwitch  DataPortOrder=Zero-based contiguous  Inputs=5  zeroidx=on
  MinMax : MinMax  Function=max  Inputs=2
  Peak trq max - Regen : Lookup  InputValues=mot.plant.init.regen.trq_max.idx1_spd  Table=mot.plant.init.regen.trq_max.map  LookUpMeth=Interpolation-Use End Values  SaturateOnIntegerOverflow=on
  Regen Trq Derating1 : Lookup_n-D  NumberOfTableDimensions=1  BreakpointsForDimension1=[0 10 11 200]  Table=[0 0.5 1 1]  ExtrapMethod=Clip  UseLastTableValue=on  InternalRulePriority=Speed  RndMeth=Simplest  InputSameDT=on
  Regen_derat_overri : Constant  Value=0
  Regen_derat_value : Constant  Value=0.5
  Switch : Switch  Criteria=u2 > Threshold
  limit to 100Nm : Saturate  UpperLimit=0  LowerLimit=-100
  T : Outport
  wires:
  MinMax/1 -> [TrqCalc]
  IntdAxleTrq/1 -> MinMax/1
  Regen_derat_value/1 -> Switch/1
  Switch/1 -> Divide/3
  Regen_derat_overri/1 -> Switch/2
  Regen Trq Derating1/1 -> Switch/3
  Divide2/1 -> MinMax/2  "motor"
  TransRatio/1 -> Divide2/3
  limit to 100Nm/1 -> Divide2/2
  Constant2/1 -> Divide2/1
  Peak trq max - Regen/1 -> Divide/2
  MotSpeed/1 -> Peak trq max - Regen/1  "RPM"
  [TrqCalc] -> Index Vector/5  "N"
  Constant1/1 -> Index Vector/3  "P"
  Constant/1 -> Index Vector/2  "Between Ranges"
  Index Vector/1 -> T/1
  [TrqCalc] -> Index Vector/6  "D"
  [TrqCalc] -> Index Vector/4  "R"
  ShftLvrPos/1 -> Index Vector/1
  VehSpd/1 -> Regen Trq Derating1/1
  Divide/1 -> limit to 100Nm/1
  "% to 1 "/1 -> Divide/1
  BPP/1 -> "% to 1 "/1

== system Clutchless_P2_Parallel/Clutchless_HSC/HSC/Powertrain Manager/Torque Distribution/Supervisory  Control  Logic/VehReady.CS_Mode.Engine_Charge.Brake_mode1.MotTrqCalc2 ==
  note: Regenerative braking:
      | Regenerative braking should be allowed under specific chassis speed:
      | chas_spd_below_no_regen= 1.5;
      | chas_spd_above_full_regen = 3;
      | ess_soc_above_regen_forbidden = .92;  % ESS SOC above which regen braking is forbidden
      | ess_soc_above_regen_allowed = .9;% ESS SOC above which regen braking is allowed
  ShftLvrPos : Inport
  TransRatio : Inport  Port=2
  f : TriggerPort  TriggerType=function-call  VariantControl=Variant
      settings: CopyFcn=Stateflow.SLINSF.SimulinkMan.removeBlockPreDeleteFcn  PreDeleteFcn=Stateflow.SLINSF.SimulinkMan.unsafePredeleteFcn
  Constant : Constant  Value=0
  Constant1 : Constant  Value=0
  Constant2 : Constant  Value=fd.plant.init.ratio
  Divide2 : Product  Inputs=***
  Idle_torque_Regen : Constant  Value=0
  Index Vector : MultiPortSwitch  DataPortOrder=Zero-based contiguous  Inputs=5  zeroidx=on
  T : Outport
  wires:
  Idle_torque_Regen/1 -> Divide2/2
  Divide2/1 -> [TrqCalc]  "motor"
  TransRatio/1 -> Divide2/3
  Constant2/1 -> Divide2/1
  [TrqCalc] -> Index Vector/5  "N"
  Constant1/1 -> Index Vector/3  "P"
  Constant/1 -> Index Vector/2  "Between Ranges"
  Index Vector/1 -> T/1
  [TrqCalc] -> Index Vector/6  "D"
  [TrqCalc] -> Index Vector/4  "R"
  ShftLvrPos/1 -> Index Vector/1

== system Clutchless_P2_Parallel/Clutchless_HSC/HSC/Powertrain Manager/Torque Distribution/Supervisory  Control  Logic/VehReady.CS_Mode.Engine_Charge.Drive_Mode.EngTrq2EngApp ==
  Trq : Inport
  TransRatio : Inport  Port=2
  f : TriggerPort  TriggerType=function-call  VariantControl=Variant
      settings: CopyFcn=Stateflow.SLINSF.SimulinkMan.removeBlockPreDeleteFcn  PreDeleteFcn=Stateflow.SLINSF.SimulinkMan.unsafePredeleteFcn
  0-100% : Saturate  UpperLimit=100  LowerLimit=0
  Compare To Constant : simulink/Logic and Bit Operations/Compare To Constant  relop===  const=0  OutDataTypeStr=boolean
  Constant1 : Constant  Value=eps
  Constant5 : Constant  Value=fd.plant.init.ratio
  Divide1 : Product  Inputs=*//
  EngTrq2EngAPP : Lookup_n-D  Commented=on  NumberOfTableDimensions=1  BreakpointsForDimension1=[0:1:230]  Table="[-0.950562242591810\t-0.861179388327002\t-0.757792747831397\t-0.640901927898975\t-0.511000095283862\t-0.368573976700328\t-0.214103858822793\t-0.0480635882858183\t0.129079428315885\t0.316864224427463\t0.514836273533913\t0.722547489160089\t0.939556224870697\t1.16542727427030\t1.39973187100331\t1.64204768875400\t1.89195884124648\t2.14905588224475\t2.41293580555262\t2.68320204501379\t2.95946447451180\t3.24133940797003\t3.52844959935174\t3.82042424266002\t4.11689897193784\t4.41751586126800\t4.72192342477317\t5.02977661661586\t5.34073683099846\t5.65447190216317\t5.97065610439209\t6.28897015200715\t6.60910119937013\t6.93074284088268\t7.25359511098630\t7.57736448416234\t7.90176387493200\t8.22651263785634\t8.55133656753627\t8.87596789861257\t9.20014530576584\t9.52361390371657\t9.84612524722509\t10.1674373310916\t10.4873145901561\t10.8055278992985\t11.1218545734385\t11.4360783675358\t11.7479894765898\t12.0573845356398\t12.3640666197649\t12.6678452440843\t12.9685363637566\t13.2659623739808\t13.5599521099953\t13.8503408470787\t14.1369703005491\t14.4196886257647\t14.6983504181235\t14.9728167130634\t15.2429549860620\t15.5086391526369\t15.7697495683456\t16.0261730287853\t16.2778027695931\t16.5245384664460\t16.7662862350608\t17.0029586311942\t17.2344746506427\t17.4607597292427\t17.6817457428705\t17.8973710074422\t18.1075802789137\t18.3123247532808\t18.5115620665792\t18.7052562948843\t18.8933779543117\t19.0759040010164\t19.2528178311935\t19.4241092810781\t19.5897746269448\t19.7498165851084\t19.9042443119232\t20.0530734037837\t20.1963258971241\t20.3340302684184\t20.4662214341804\t20.5929407509641\t20.7142360153630\t20.8301614640105\t20.9407777735800\t21.0461520607847\t21.1463578823776\t21.2414752351516\t21.3315905559394\t21.4167967216136\t21.4971930490867\t21.5728852953111\t21.6439856572787\t21.7106127720217\t21.7728917166119\t21.8309540081611\t21.8849376038208\t21.9349869007824\t21.9812527362772\t22.0238923875764\t22.0630695719909\t22.0989544468717\t22.1317236096093\t22.1615600976344\t22.1886533884173\t22.2131993994684\t22.2354004883376\t22.2554654526151\t22.2736095299306\t22.2900543979538\t22.3050281743942\t22.3187654170013\t22.3315071235641\t22.3435007319120\t22.3550001199137\t22.3662656054781\t22.3775639465539\t22.3891683411296\t22.4013584272335\t22.4144202829338\t22.4286464263386\t22.4443358155959\t22.4617938488934\t22.4813323644587\t22.5032696405595\t22.5279303955028\t22.5556457876361\t22.5867534153463\t22.6215973170604\t22.6605279712450\t22.7039022964069\t22.7520836510924\t22.8054418338880\t22.8643530834197\t22.9292000783536\t23.0003719373956\t23.0782642192915\t23.1632789228268\t23.2558244868269\t23.3563157901571\t23.4651741517227\t23.5828273304686\t23.7097095253797\t23.8462613754808\t23.9929299598362\t24.1501687975506\t24.3184378477682\t24.4982035096730\t24.6899386224892\t24.8941224654804\t25.1112407579505\t25.3417856592430\t25.5862557687413\t25.8451561258686\t26.1189982100880\t26.4082999409026\t26.7135856778550\t27.0353862205281\t27.3742388085443\t27.7306871215661\t28.1052812792955\t28.4985778414748\t28.9111398078859\t29.3435366183506\t29.7963441527305\t30.2701447309271\t30.7655271128819\t31.2830864985759\t31.8234245280303\t32.3871492813060\t32.9748752785038\t33.5872234797643\t34.2248212852680\t34.8883025352352\t35.5783075099261\t36.2954829296408\t37.0404819547192\t37.8139641855409\t38.6165956625258\t39.4490488661331\t40.3120027168621\t41.2061425752523\t42.1321602418824\t43.0907539573713\t44.0826284023780\t45.1084946976008\t46.1690704037782\t47.2650795216887\t48.3972524921501\t49.5663261960208\t50.7730439541983\t52.0181555276205\t53.3024171172650\t54.6265913641491\t55.9914473493301\t57.3977605939052\t58.8463130590113\t60.3378931458253\t61.8732956955639\t63.4533219894835\t65.0787797488808\t66.7504831350916\t68.4692527494924\t70.2359156334991\t72.0513052685674\t73.9162615761929\t75.8316309179113\t77.7982660952979\t79.8170263499681\t81.8887773635766\t84.0143912578187\t86.1947465944290\t88.4307283751822\t90.7232280418928\t93.0731434764153\t95.4813790006436\t97.9488453765121\t100\t100\t100\t100\t100\t100\t100\t100]"  ExtrapMethod=Clip  UseLastTableValue=on  InternalRulePriority=Speed  RndMeth=Simplest  InputSameDT=on
  EngTrq2EngAPP_Linear : Lookup_n-D  NumberOfTableDimensions=1  BreakpointsForDimension1=[0:1:250]  Table=[0:0.4:100]  ExtrapMethod=Clip  UseLastTableValue=on  InternalRulePriority=Speed  RndMeth=Simplest  InputSameDT=on
  Switch : Switch  Criteria=u2 > Threshold
  APP : Outport
  wires:
  EngTrq2EngAPP_Linear/1 -> 0-100%/1  "EngTrq2EngAPP_CS"
  0-100%/1 -> APP/1
  TransRatio/1 -> Compare To Constant/1, Switch/3
  Divide1/1 -> EngTrq2EngAPP_Linear/1
  Switch/1 -> Divide1/3
  Constant1/1 -> Switch/1
  Compare To Constant/1 -> Switch/2
  Constant5/1 -> Divide1/2
  Trq/1 -> Divide1/1  "EngAxlTrqReq_CS"

== system Clutchless_P2_Parallel/Clutchless_HSC/HSC/Powertrain Manager/Torque Distribution/Supervisory  Control  Logic/VehReady.CS_Mode.Engine_Charge.Drive_Mode.EngTrqCalc ==
  EngSpeed : Inport
  APP : Inport  Port=2
  VehSpd : Inport  Port=3
  ShftLvrPos : Inport  Port=4
  DrvIntdAxleTrq : Inport  Port=5
  TransRatio : Inport  Port=6
  SOC : Inport  Port=7
  f : TriggerPort  TriggerType=function-call  VariantControl=Variant
      settings: CopyFcn=Stateflow.SLINSF.SimulinkMan.removeBlockPreDeleteFcn  PreDeleteFcn=Stateflow.SLINSF.SimulinkMan.unsafePredeleteFcn
  APP Derating : Lookup_n-D  NumberOfTableDimensions=1  BreakpointsForDimension1=[0 1 2 3 5 7]  Table=[0 0.1 0.3 0.5 0.7 1]  ExtrapMethod=Clip  UseLastTableValue=on  InternalRulePriority=Speed  RndMeth=Simplest  InputSameDT=on
  Constant : Constant  Value=0
  Constant1 : Constant  Value=0
  Constant3 : Constant  Value=fd.plant.init.ratio
  Divide : Product  Inputs=***
  Divide2 : Product  Inputs=***
  EngOptmTrq_Original : Lookup_n-D  NumberOfTableDimensions=1  BreakpointsForDimension1=[1550 1650 1850 2050 2350 2650 2950 3150 3250 3350]  Table="[154.020912669576\t173.623574282068\t180.662367834043\t186.327738253926\t182.858870786433\t180.175407273844\t178.037732950256\t181.891363533595\t190.985931710274\t199.537540592824]"  ExtrapMethod=Clip  UseLastTableValue=on  InternalRulePriority=Speed  RndMeth=Simplest  InputSameDT=on
  Engine Max Trq : Lookup_n-D  NumberOfTableDimensions=1  BreakpointsForDimension1="[600\t800\t1000\t1200\t1400\t1600\t1800\t2000\t2200\t2400\t2600\t2800\t3000\t3200\t3400\t3600\t3800\t4000\t4250\t4500\t4750\t5000\t5250\t5500\t5750\t6000\t6250\t6500]"  Table="[83.7900000000000\t136.760000000000\t140\t152.010000000000\t171.590000000000\t185.900000000000\t198.400000000000\t197.360000000000\t200.550000000000\t202.260000000000\t215.080000000000\t204.810000000000\t204.520000000000\t208.100000000000\t211.520000000000\t210.560000000000\t214.100000000000\t213.470000000000\t208.730000000000\t208.430000000000\t208.670000000000\t231.210000000000\t228.310000000000\t225.330000000000\t220.520000000000\t211.210000000000\t204.190000000000\t151.770000000000]"  ExtrapMethod=Clip  UseLastTableValue=on  InternalRulePriority=Speed  RndMeth=Simplest  InputSameDT=on
  MinMax : MinMax  Function=max  Inputs=2
  SOC Window Estimation : Subsystem
  Shifter : MultiPortSwitch  DataPortOrder=Zero-based contiguous  Inputs=5  zeroidx=on
  Switch : Switch  Criteria=u2 > Threshold
  VehSpd Derating : Lookup_n-D  NumberOfTableDimensions=1  BreakpointsForDimension1=[0 2 5]  Table=[0 0.5 1]  ExtrapMethod=Clip  UseLastTableValue=on  InternalRulePriority=Speed  RndMeth=Simplest  InputSameDT=on
  Trq : Outport
  EngActTRq : Outport  Port=2
  wires:
  MinMax/1 -> [TrqCalc]  "EngAxlTrqReq_CS"
  Constant3/1 -> Divide2/3
  TransRatio/1 -> Divide2/1
  EngOptmTrq_Original/1 -> Switch/3
  Engine Max Trq/1 -> Switch/1
  SOC Window Estimation/1(Out1) -> Switch/2
  SOC/1 -> SOC Window Estimation/1(SOC)
  Switch/1 -> Divide/1  "EngTrqAvl_CS"
  DrvIntdAxleTrq/1 -> MinMax/1  "DrvIntdAxlTrq_CS"
  Divide2/1 -> MinMax/2, EngActTRq/1  "EngAxlTrqAvl_CS"
  Divide/1 -> Divide2/2
  Shifter/1 -> Trq/1
  [TrqCalc] -> Shifter/5  "N"
  Constant1/1 -> Shifter/3  "P"
  Constant/1 -> Shifter/2  "Between Ranges"
  [TrqCalc] -> Shifter/6  "D"
  [TrqCalc] -> Shifter/4  "R"
  ShftLvrPos/1 -> Shifter/1
  VehSpd Derating/1 -> Divide/3  "VehSpeedDerating_CS"
  VehSpd/1 -> VehSpd Derating/1
  APP Derating/1 -> Divide/2  "APPDerating_CS"
  APP/1 -> APP Derating/1
  EngSpeed/1 -> Engine Max Trq/1, EngOptmTrq_Original/1

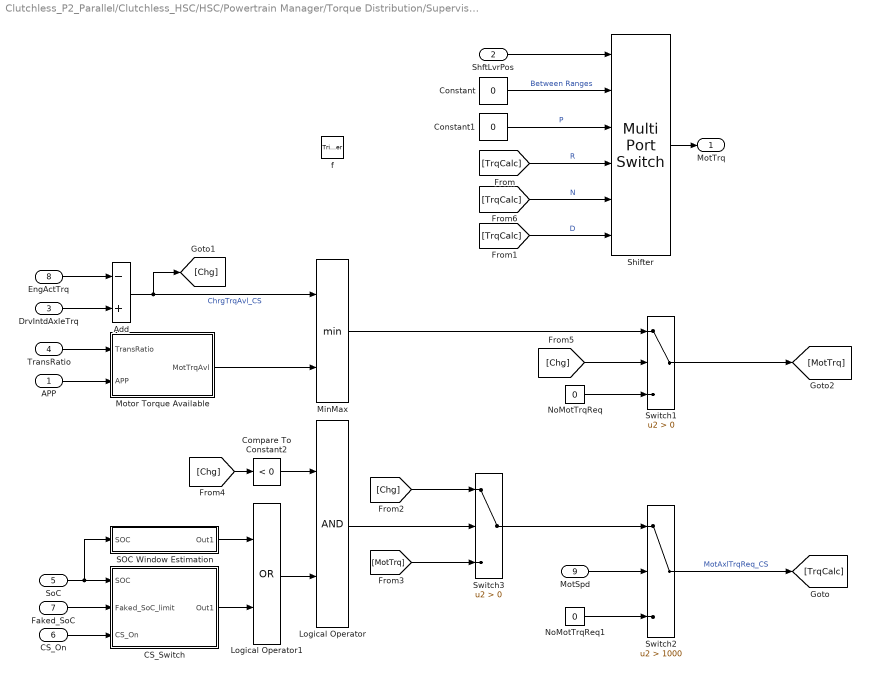
== system Clutchless_P2_Parallel/Clutchless_HSC/HSC/Powertrain Manager/Torque Distribution/Supervisory  Control  Logic/VehReady.CS_Mode.Engine_Charge.Drive_Mode.MotTrqCalc ==
  APP : Inport
  ShftLvrPos : Inport  Port=2
  DrvIntdAxleTrq : Inport  Port=3
  TransRatio : Inport  Port=4
  SoC : Inport  Port=5
  CS_On : Inport  Port=6
  Faked_SoC : Inport  Port=7
  EngActTrq : Inport  Port=8
  MotSpd : Inport  Port=9
  f : TriggerPort  TriggerType=function-call  VariantControl=Variant
      settings: CopyFcn=Stateflow.SLINSF.SimulinkMan.removeBlockPreDeleteFcn  PreDeleteFcn=Stateflow.SLINSF.SimulinkMan.unsafePredeleteFcn
  Add : Sum  Inputs=-+
  CS_Switch : Subsystem
  Compare To Constant2 : simulink/Logic and Bit Operations/Compare To Constant  relop=<  const=0  OutDataTypeStr=boolean
  Constant : Constant  Value=0
  Constant1 : Constant  Value=0
  Logical Operator : Logic  AllPortsSameDT=off  OutDataTypeStr=boolean
  Logical Operator1 : Logic  Operator=OR  AllPortsSameDT=off  OutDataTypeStr=boolean
  MinMax : MinMax  Inputs=2
  Motor Torque Available : Subsystem
  NoMotTrqReq : Constant  Value=0
  NoMotTrqReq1 : Constant  Value=0
  SOC Window Estimation : Subsystem
  Shifter : MultiPortSwitch  DataPortOrder=Zero-based contiguous  Inputs=5  zeroidx=on
  Switch1 : Switch  Criteria=u2 > Threshold
  Switch2 : Switch  Criteria=u2 > Threshold  Threshold=1000
  Switch3 : Switch  Criteria=u2 > Threshold
  MotTrq : Outport
  wires:
  [Chg] -> Switch1/2
  MotSpd/1 -> Switch2/2
  Motor Torque Available/1(MotTrqAvl) -> MinMax/2
  APP/1 -> Motor Torque Available/2(APP)
  TransRatio/1 -> Motor Torque Available/1(TransRatio)
  [Chg] -> Compare To Constant2/1
  [MotTrq] -> Switch3/3
  Switch1/1 -> [MotTrq]
  EngActTrq/1 -> Add/1
  Switch2/1 -> [TrqCalc]  "MotAxlTrqReq_CS"
  NoMotTrqReq1/1 -> Switch2/3
  CS_Switch/1(Out1) -> Logical Operator1/2
  CS_On/1 -> CS_Switch/3(CS_On)
  Faked_SoC/1 -> CS_Switch/2(Faked_SoC_limit)
  SOC Window Estimation/1(Out1) -> Logical Operator1/1
  Logical Operator1/1 -> Logical Operator/2
  Switch3/1 -> Switch2/1
  [Chg] -> Switch3/1
  Logical Operator/1 -> Switch3/2
  Compare To Constant2/1 -> Logical Operator/1
  NoMotTrqReq/1 -> Switch1/3
  MinMax/1 -> Switch1/1
  Add/1 -> MinMax/1, [Chg]  "ChrgTrqAvl_CS"
  SoC/1 -> CS_Switch/1(SOC), SOC Window Estimation/1(SOC)
  DrvIntdAxleTrq/1 -> Add/2
  Shifter/1 -> MotTrq/1
  [TrqCalc] -> Shifter/5  "N"
  Constant1/1 -> Shifter/3  "P"
  Constant/1 -> Shifter/2  "Between Ranges"
  [TrqCalc] -> Shifter/6  "D"
  [TrqCalc] -> Shifter/4  "R"
  ShftLvrPos/1 -> Shifter/1
